simulink model "sampleModel7293"  (R2018a)
settings: Solver=VariableStepAuto  StartTime=0.0  StopTime=10.0  RelTol=1e-3
undefined symbols (not defined in the file): DiscIntNeverNeededParam
libraries: simulink x367
(part 3 of 7)

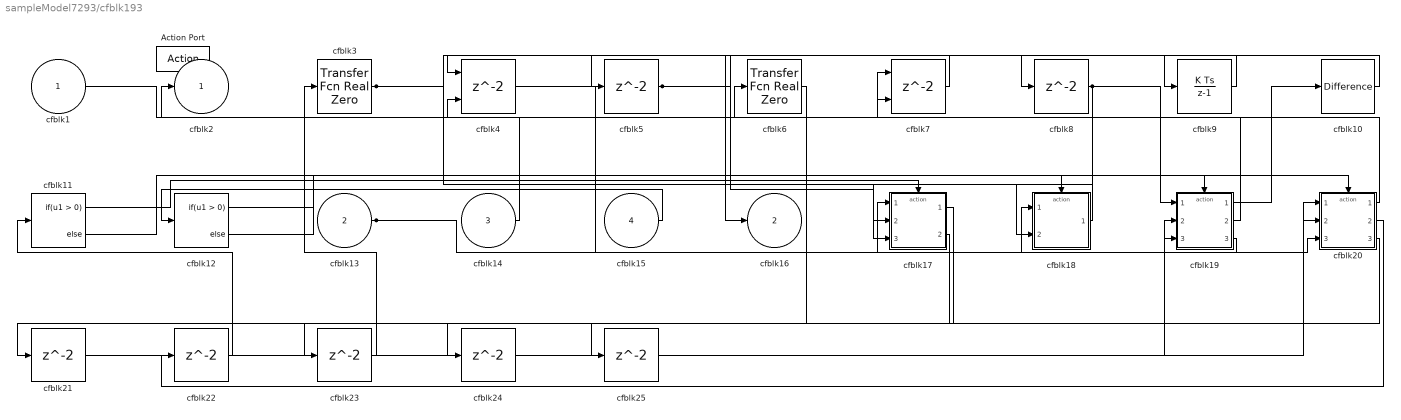
== system sampleModel7293/cfblk193 ==
  cfblk1 : Inport
  cfblk13 : Inport  Port=2
  cfblk14 : Inport  Port=3
  cfblk15 : Inport  Port=4
  Action Port : ActionPort  ActionType=else
  cfblk10 : simulink/Discrete/Difference  ICPrevInput=0.0  OutMin=[]  OutMax=[]  OutDataTypeStr=Inherit: Inherit via back propagation  OutDataType=fixdt(1, 16)  OutScaling=2^-10  DoSatur=off
  cfblk11 : If  SampleTime=1
  cfblk12 : If  SampleTime=1
  cfblk17 : Subsystem  TreatAsAtomicUnit=on
  cfblk18 : Subsystem  TreatAsAtomicUnit=on
  cfblk19 : Subsystem  TreatAsAtomicUnit=on
  cfblk20 : Subsystem  TreatAsAtomicUnit=on
  cfblk{5,8,21..25} (7 alike) : Delay
  cfblk3 : simulink/Discrete/Transfer Fcn Real Zero  ZeroZ=0.75  ICPrevInput=0.0  DoSatur=off
      settings: SourceProductName=Simulink  SourceProductBaseCode=SL
  cfblk4 : Delay  ShowEnablePort=on
      settings: InputPortMap=u0,e6
  cfblk6 : simulink/Discrete/Transfer Fcn Real Zero  ZeroZ=0.75  ICPrevInput=0.0  DoSatur=off
      settings: SourceProductName=Simulink  SourceProductBaseCode=SL
  cfblk7 : Delay  ShowEnablePort=on
      settings: InputPortMap=u0,e6
  cfblk9 : DiscreteIntegrator  SampleTime=-1  ICPrevOutput=DiscIntNeverNeededParam  ICPrevScaledInput=DiscIntNeverNeededParam
  cfblk2 : Outport
  cfblk16 : Outport  Port=2
  wires:
  cfblk18/1(cfblk2) -> cfblk6/1
  cfblk7/1 -> cfblk16/1
  cfblk9/1 -> cfblk4/1
  cfblk19/1(cfblk2) -> cfblk10/1
  cfblk20/1(cfblk2) -> cfblk7/1
  cfblk14/1 -> cfblk4/2
  cfblk4/1 -> cfblk17/1(cfblk1)
  cfblk10/1 -> cfblk9/1
  cfblk5/1 -> cfblk8/1, cfblk17/2(cfblk12)
  cfblk15/1 -> cfblk12/1
  cfblk19/2(cfblk15) -> cfblk2/1
  cfblk1/1 -> cfblk7/2
  cfblk8/1 -> cfblk19/1(cfblk1), cfblk17/3(cfblk13)
  cfblk3/1 -> cfblk5/1, cfblk18/2(cfblk11)
  cfblk13/1 -> cfblk19/2(cfblk13), cfblk20/3(cfblk14)
  cfblk19/3(cfblk16) -> cfblk18/1(cfblk1)
  cfblk11/1 -> cfblk17/Action
  cfblk11/2 -> cfblk18/Action
  cfblk12/1 -> cfblk19/Action
  cfblk12/2 -> cfblk20/Action
  cfblk17/1(cfblk2) -> cfblk21/1
  cfblk21/1 -> cfblk20/1(cfblk1)
  cfblk20/2(cfblk15) -> cfblk22/1
  cfblk22/1 -> cfblk11/1
  cfblk6/1 -> cfblk23/1
  cfblk23/1 -> cfblk3/1
  cfblk20/3(cfblk16) -> cfblk24/1
  cfblk24/1 -> cfblk19/3(cfblk14)
  cfblk17/2(cfblk14) -> cfblk25/1
  cfblk25/1 -> cfblk20/2(cfblk13)

== system sampleModel7293/cfblk194 ==
  cfblk1 : Inport
  Action Port : ActionPort  ActionType=then
  cfblk3 : Delay
  cfblk4 : simulink/Continuous/PID Controller  Controller=PID  TimeDomain=Discrete-time  SampleTime=-1  IntegratorMethod=Forward Euler  FilterMethod=Forward Euler  Form=Parallel  UseFilter=on  ControllerParametersSource=internal  P=1  I=1  D=0  N=100  InitialConditionSource=internal  InitialConditionForIntegrator=0  InitialConditionForFilter=0  ExternalReset=none  LimitOutput=off  UpperSaturationLimit=inf  LowerSaturationLimit=-inf  LinearizeAsGain=off  AntiWindupMode=none  Kb=1  TrackingMode=off  Kt=1  PParamMin=[]  PParamMax=[]  IParamMin=[]  IParamMax=[]  DParamMin=[]  DParamMax=[]  NParamMin=[]  NParamMax=[]  KbParamMin=[]  KbParamMax=[]  KtParamMin=[]  KtParamMax=[]  POutMin=[]  POutMax=[]  IOutMin=[]  IOutMax=[]  DOutMin=[]  DOutMax=[]  NOutMin=[]  NOutMax=[]  KbOutMin=[]  KbOutMax=[]  KtOutMin=[]  KtOutMax=[]  IntegratorOutMin=[]  IntegratorOutMax=[]  FilterOutMin=[]  FilterOutMax=[]  SumOutMin=[]  SumOutMax=[]  SumI1OutMin=[]  SumI1OutMax=[]  SumI2OutMin=[]  SumI2OutMax=[]  SumI3OutMin=[]  SumI3OutMax=[]  SumDOutMin=[]  SumDOutMax=[]  SaturationOutMin=[]  SaturationOutMax=[]  IntegratorContinuousStateAttributes=''  IntegratorStateMustResolveToSignalObject=off  IntegratorRTWStateStorageClass=Auto  FilterContinuousStateAttributes=''  FilterStateMustResolveToSignalObject=off  FilterRTWStateStorageClass=Auto  DifferentiatorICPrevScaledInput=0  DifferentiatorOutMin=[]  DifferentiatorOutMax=[]  InitialConditionSetting=State (most efficient)
  cfblk5 : UnitDelay  SampleTime=-1
  cfblk6 : DiscreteTransferFcn
  cfblk7 : Delay  ShowEnablePort=on
      settings: InputPortMap=u0,e6
  cfblk8 : Delay
  cfblk2 : Outport
  wires:
  cfblk4/1 -> cfblk2/1
  cfblk3/1 -> cfblk6/1
  cfblk1/1 -> cfblk5/1
  cfblk6/1 -> cfblk7/2, cfblk8/1
  cfblk5/1 -> cfblk7/1
  cfblk7/1 -> cfblk4/1
  cfblk8/1 -> cfblk3/1

== system sampleModel7293/cfblk195 ==
  cfblk1 : Inport
  cfblk7 : Inport  Port=2
  Action Port : ActionPort  ActionType=else
  cfblk{10..13} (4 alike) : Delay
  cfblk3 : Delay  ShowEnablePort=on
      settings: InputPortMap=u0,e6
  cfblk4 : simulink/Discrete/Difference  ICPrevInput=0.0  OutMin=[]  OutMax=[]  OutDataTypeStr=Inherit: Inherit via back propagation  OutDataType=fixdt(1, 16)  OutScaling=2^-10  DoSatur=off
  cfblk5 : simulink/Discrete/Transfer Fcn Lead or Lag  PoleZ=0.95  ZeroZ=0.75  ICPrevOutput=0.0  ICPrevInput=0.0  DoSatur=off
      settings: SourceProductName=Simulink  SourceProductBaseCode=SL
  cfblk6 : If  SampleTime=1
  cfblk8 : Subsystem  TreatAsAtomicUnit=on
  cfblk9 : Subsystem  TreatAsAtomicUnit=on
  cfblk2 : Outport
  wires:
  cfblk3/1 -> cfblk5/1, cfblk13/1
  cfblk9/1(cfblk2) -> cfblk8/1(cfblk1)
  cfblk5/1 -> cfblk2/1
  cfblk8/1(cfblk2) -> cfblk4/1, cfblk10/1, cfblk12/1
  cfblk9/2(cfblk14) -> cfblk8/2(cfblk11)
  cfblk7/1 -> cfblk3/1
  cfblk1/1 -> cfblk9/2(cfblk11)
  cfblk9/3(cfblk15) -> cfblk8/3(cfblk12), cfblk3/2
  cfblk6/1 -> cfblk8/Action
  cfblk6/2 -> cfblk9/Action
  cfblk10/1 -> cfblk9/1(cfblk1)
  cfblk4/1 -> cfblk11/1
  cfblk11/1 -> cfblk6/1
  cfblk12/1 -> cfblk9/4(cfblk13)
  cfblk13/1 -> cfblk9/3(cfblk12)

== system sampleModel7293/cfblk196 ==
  cfblk1 : Inport
  cfblk9 : Inport  Port=2
  cfblk10 : Inport  Port=3
  Action Port : ActionPort  ActionType=then
  cfblk11 : Subsystem  TreatAsAtomicUnit=on
  cfblk12 : Subsystem  TreatAsAtomicUnit=on
  cfblk13 : Delay
  cfblk14 : Delay
  cfblk3 : simulink/Continuous/PID Controller  Controller=PID  TimeDomain=Discrete-time  SampleTime=-1  IntegratorMethod=Forward Euler  FilterMethod=Forward Euler  Form=Parallel  UseFilter=on  ControllerParametersSource=internal  P=1  I=1  D=0  N=100  InitialConditionSource=internal  InitialConditionForIntegrator=0  InitialConditionForFilter=0  ExternalReset=none  LimitOutput=off  UpperSaturationLimit=inf  LowerSaturationLimit=-inf  LinearizeAsGain=off  AntiWindupMode=none  Kb=1  TrackingMode=off  Kt=1  PParamMin=[]  PParamMax=[]  IParamMin=[]  IParamMax=[]  DParamMin=[]  DParamMax=[]  NParamMin=[]  NParamMax=[]  KbParamMin=[]  KbParamMax=[]  KtParamMin=[]  KtParamMax=[]  POutMin=[]  POutMax=[]  IOutMin=[]  IOutMax=[]  DOutMin=[]  DOutMax=[]  NOutMin=[]  NOutMax=[]  KbOutMin=[]  KbOutMax=[]  KtOutMin=[]  KtOutMax=[]  IntegratorOutMin=[]  IntegratorOutMax=[]  FilterOutMin=[]  FilterOutMax=[]  SumOutMin=[]  SumOutMax=[]  SumI1OutMin=[]  SumI1OutMax=[]  SumI2OutMin=[]  SumI2OutMax=[]  SumI3OutMin=[]  SumI3OutMax=[]  SumDOutMin=[]  SumDOutMax=[]  SaturationOutMin=[]  SaturationOutMax=[]  IntegratorContinuousStateAttributes=''  IntegratorStateMustResolveToSignalObject=off  IntegratorRTWStateStorageClass=Auto  FilterContinuousStateAttributes=''  FilterStateMustResolveToSignalObject=off  FilterRTWStateStorageClass=Auto  DifferentiatorICPrevScaledInput=0  DifferentiatorOutMin=[]  DifferentiatorOutMax=[]  InitialConditionSetting=State (most efficient)
  cfblk4 : simulink/Discrete/Transfer Fcn Lead or Lag  PoleZ=0.95  ZeroZ=0.75  ICPrevOutput=0.0  ICPrevInput=0.0  DoSatur=off
      settings: SourceProductName=Simulink  SourceProductBaseCode=SL
  cfblk5 : Delay  ShowEnablePort=on
      settings: InputPortMap=u0,e6
  cfblk6 : DiscreteStateSpace  SampleTime=-1
  cfblk7 : DiscreteIntegrator  SampleTime=-1  ICPrevOutput=DiscIntNeverNeededParam  ICPrevScaledInput=DiscIntNeverNeededParam
  cfblk8 : If  SampleTime=1
  cfblk2 : Outport
  wires:
  cfblk12/1(cfblk2) -> cfblk2/1
  cfblk3/1 -> cfblk4/1
  cfblk6/1 -> cfblk7/1
  cfblk10/1 -> cfblk3/1
  cfblk12/2(cfblk12) -> cfblk6/1
  cfblk4/1 -> cfblk12/1(cfblk1)
  cfblk9/1 -> cfblk5/1
  cfblk1/1 -> cfblk11/2(cfblk10), cfblk11/3(cfblk11)
  cfblk11/1(cfblk2) -> cfblk5/2
  cfblk8/1 -> cfblk11/Action
  cfblk8/2 -> cfblk12/Action
  cfblk5/1 -> cfblk13/1
  cfblk13/1 -> cfblk8/1
  cfblk7/1 -> cfblk14/1
  cfblk14/1 -> cfblk11/1(cfblk1)

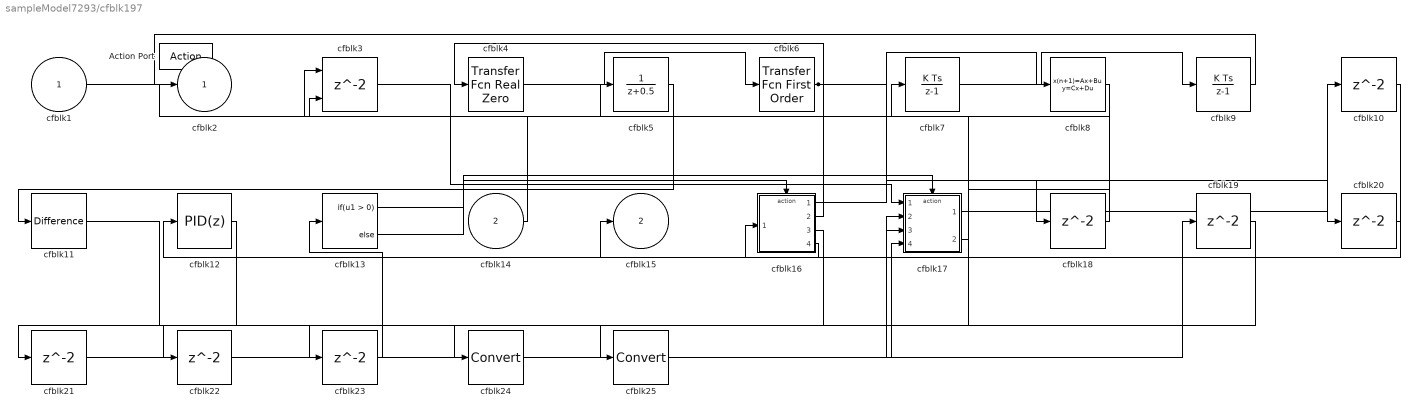
== system sampleModel7293/cfblk197 ==
  cfblk1 : Inport
  cfblk14 : Inport  Port=2
  Action Port : ActionPort  ActionType=else
  cfblk{10,18..23} (7 alike) : Delay
  cfblk11 : simulink/Discrete/Difference  ICPrevInput=0.0  OutMin=[]  OutMax=[]  OutDataTypeStr=Inherit: Inherit via back propagation  OutDataType=fixdt(1, 16)  OutScaling=2^-10  DoSatur=off
  cfblk12 : simulink/Continuous/PID Controller  Controller=PID  TimeDomain=Discrete-time  SampleTime=-1  IntegratorMethod=Forward Euler  FilterMethod=Forward Euler  Form=Parallel  UseFilter=on  ControllerParametersSource=internal  P=1  I=1  D=0  N=100  InitialConditionSource=internal  InitialConditionForIntegrator=0  InitialConditionForFilter=0  ExternalReset=none  LimitOutput=off  UpperSaturationLimit=inf  LowerSaturationLimit=-inf  LinearizeAsGain=off  AntiWindupMode=none  Kb=1  TrackingMode=off  Kt=1  PParamMin=[]  PParamMax=[]  IParamMin=[]  IParamMax=[]  DParamMin=[]  DParamMax=[]  NParamMin=[]  NParamMax=[]  KbParamMin=[]  KbParamMax=[]  KtParamMin=[]  KtParamMax=[]  POutMin=[]  POutMax=[]  IOutMin=[]  IOutMax=[]  DOutMin=[]  DOutMax=[]  NOutMin=[]  NOutMax=[]  KbOutMin=[]  KbOutMax=[]  KtOutMin=[]  KtOutMax=[]  IntegratorOutMin=[]  IntegratorOutMax=[]  FilterOutMin=[]  FilterOutMax=[]  SumOutMin=[]  SumOutMax=[]  SumI1OutMin=[]  SumI1OutMax=[]  SumI2OutMin=[]  SumI2OutMax=[]  SumI3OutMin=[]  SumI3OutMax=[]  SumDOutMin=[]  SumDOutMax=[]  SaturationOutMin=[]  SaturationOutMax=[]  IntegratorContinuousStateAttributes=''  IntegratorStateMustResolveToSignalObject=off  IntegratorRTWStateStorageClass=Auto  FilterContinuousStateAttributes=''  FilterStateMustResolveToSignalObject=off  FilterRTWStateStorageClass=Auto  DifferentiatorICPrevScaledInput=0  DifferentiatorOutMin=[]  DifferentiatorOutMax=[]  InitialConditionSetting=State (most efficient)
  cfblk13 : If  SampleTime=1
  cfblk16 : Subsystem  TreatAsAtomicUnit=on
  cfblk17 : Subsystem  TreatAsAtomicUnit=on
  cfblk24 : DataTypeConversion
  cfblk25 : DataTypeConversion
  cfblk3 : Delay  ShowEnablePort=on
      settings: InputPortMap=u0,e6
  cfblk4 : simulink/Discrete/Transfer Fcn Real Zero  ZeroZ=0.75  ICPrevInput=0.0  DoSatur=off
      settings: SourceProductName=Simulink  SourceProductBaseCode=SL
  cfblk5 : DiscreteTransferFcn
  cfblk6 : simulink/Discrete/Transfer Fcn First Order  PoleZ=0.95  ICPrevOutput=0.0  DoSatur=off
      settings: SourceProductName=Simulink
  cfblk7 : DiscreteIntegrator  SampleTime=-1  ICPrevOutput=DiscIntNeverNeededParam  ICPrevScaledInput=DiscIntNeverNeededParam
  cfblk8 : DiscreteStateSpace  SampleTime=-1
  cfblk9 : DiscreteIntegrator  SampleTime=-1  ICPrevOutput=DiscIntNeverNeededParam  ICPrevScaledInput=DiscIntNeverNeededParam
  cfblk2 : Outport
  cfblk15 : Outport  Port=2
  wires:
  cfblk4/1 -> cfblk6/1
  cfblk7/1 -> cfblk9/1
  cfblk16/2(cfblk11) -> cfblk4/1
  cfblk14/1 -> cfblk3/2
  cfblk10/1 -> cfblk15/1
  cfblk9/1 -> cfblk2/1
  cfblk3/1 -> cfblk17/1(cfblk1)
  cfblk17/1(cfblk2) -> cfblk10/1
  cfblk17/2(cfblk15) -> cfblk5/1
  cfblk1/1 -> cfblk7/1
  cfblk6/1 -> cfblk8/1, cfblk20/1
  cfblk5/1 -> cfblk11/1
  cfblk16/4(cfblk13) -> cfblk12/1
  cfblk13/1 -> cfblk16/Action
  cfblk13/2 -> cfblk17/Action
  cfblk16/1(cfblk2) -> cfblk18/1
  cfblk18/1 -> cfblk3/1
  cfblk20/1 -> cfblk16/1(cfblk1)
  cfblk16/3(cfblk12) -> cfblk21/1
  cfblk21/1 -> cfblk17/4(cfblk14)
  cfblk12/1 -> cfblk22/1
  cfblk22/1 -> cfblk17/3(cfblk13)
  cfblk11/1 -> cfblk23/1
  cfblk23/1 -> cfblk13/1
  cfblk19/1 -> cfblk24/1
  cfblk24/1 -> cfblk17/2(cfblk12)
  cfblk8/1 -> cfblk25/1
  cfblk25/1 -> cfblk19/1

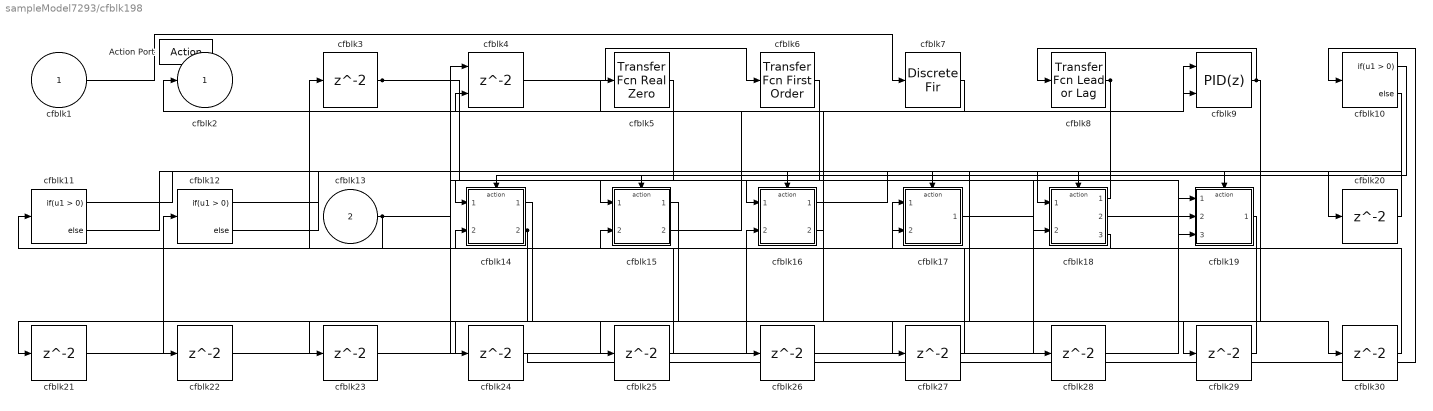
== system sampleModel7293/cfblk198 ==
  cfblk1 : Inport
  cfblk13 : Inport  Port=2
  Action Port : ActionPort  ActionType=then
  cfblk10 : If  SampleTime=1
  cfblk11 : If  SampleTime=1
  cfblk12 : If  SampleTime=1
  cfblk14 : Subsystem  TreatAsAtomicUnit=on
  cfblk15 : Subsystem  TreatAsAtomicUnit=on
  cfblk16 : Subsystem  TreatAsAtomicUnit=on
  cfblk17 : Subsystem  TreatAsAtomicUnit=on
  cfblk18 : Subsystem  TreatAsAtomicUnit=on
  cfblk19 : Subsystem  TreatAsAtomicUnit=on
  cfblk{3,20..30} (12 alike) : Delay
  cfblk4 : Delay  ShowEnablePort=on
      settings: InputPortMap=u0,e6
  cfblk5 : simulink/Discrete/Transfer Fcn Real Zero  ZeroZ=0.75  ICPrevInput=0.0  DoSatur=off
      settings: SourceProductName=Simulink  SourceProductBaseCode=SL
  cfblk6 : simulink/Discrete/Transfer Fcn First Order  PoleZ=0.95  ICPrevOutput=0.0  DoSatur=off
      settings: SourceProductName=Simulink
  cfblk7 : DiscreteFir
  cfblk8 : simulink/Discrete/Transfer Fcn Lead or Lag  PoleZ=0.95  ZeroZ=0.75  ICPrevOutput=0.0  ICPrevInput=0.0  DoSatur=off
      settings: SourceProductName=Simulink  SourceProductBaseCode=SL
  cfblk9 : simulink/Continuous/PID Controller (2DOF)  Controller=PID  TimeDomain=Discrete-time  SampleTime=-1  IntegratorMethod=Forward Euler  FilterMethod=Forward Euler  Form=Parallel  UseFilter=on  ControllerParametersSource=internal  P=1  I=1  D=0  N=100  b=1  c=1  InitialConditionSource=internal  InitialConditionForIntegrator=0  InitialConditionForFilter=0  ExternalReset=none  LimitOutput=off  UpperSaturationLimit=inf  LowerSaturationLimit=-inf  LinearizeAsGain=off  AntiWindupMode=none  Kb=1  TrackingMode=off  Kt=1  PParamMin=[]  PParamMax=[]  IParamMin=[]  IParamMax=[]  DParamMin=[]  DParamMax=[]  NParamMin=[]  NParamMax=[]  bParamMin=[]  bParamMax=[]  cParamMin=[]  cParamMax=[]  KbParamMin=[]  KbParamMax=[]  KtParamMin=[]  KtParamMax=[]  POutMin=[]  POutMax=[]  IOutMin=[]  IOutMax=[]  DOutMin=[]  DOutMax=[]  NOutMin=[]  NOutMax=[]  bOutMin=[]  bOutMax=[]  cOutMin=[]  cOutMax=[]  KbOutMin=[]  KbOutMax=[]  KtOutMin=[]  KtOutMax=[]  IntegratorOutMin=[]  IntegratorOutMax=[]  FilterOutMin=[]  FilterOutMax=[]  SumOutMin=[]  SumOutMax=[]  Sum1OutMin=[]  Sum1OutMax=[]  Sum2OutMin=[]  Sum2OutMax=[]  Sum3OutMin=[]  Sum3OutMax=[]  SumI1OutMin=[]  SumI1OutMax=[]  SumI2OutMin=[]  SumI2OutMax=[]  SumI3OutMin=[]  SumI3OutMax=[]  SumDOutMin=[]  SumDOutMax=[]  SaturationOutMin=[]  SaturationOutMax=[]  IntegratorContinuousStateAttributes=''  IntegratorStateMustResolveToSignalObject=off  IntegratorRTWStateStorageClass=Auto  FilterContinuousStateAttributes=''  FilterStateMustResolveToSignalObject=off  FilterRTWStateStorageClass=Auto  DifferentiatorICPrevScaledInput=0  DifferentiatorOutMin=[]  DifferentiatorOutMax=[]  InitialConditionSetting=State (most efficient)
  cfblk2 : Outport
  wires:
  cfblk7/1 -> cfblk2/1
  cfblk6/1 -> cfblk16/1(cfblk1)
  cfblk4/1 -> cfblk6/1
  cfblk3/1 -> cfblk18/2(cfblk14), cfblk19/3(cfblk10)
  cfblk5/1 -> cfblk14/1(cfblk1)
  cfblk9/1 -> cfblk8/1, cfblk29/1
  cfblk13/1 -> cfblk11/1, cfblk9/2, cfblk15/1(cfblk1)
  cfblk16/2(cfblk15) -> cfblk5/1
  cfblk1/1 -> cfblk7/1
  cfblk15/2(cfblk7) -> cfblk9/1
  cfblk18/1(cfblk2) -> cfblk4/2
  cfblk8/1 -> cfblk26/1, cfblk27/1
  cfblk14/2(cfblk11) -> cfblk23/1, cfblk24/1
  cfblk18/3(cfblk16) -> cfblk17/1(cfblk1)
  cfblk10/1 -> cfblk14/Action
  cfblk10/2 -> cfblk15/Action
  cfblk11/1 -> cfblk16/Action
  cfblk11/2 -> cfblk17/Action
  cfblk12/1 -> cfblk18/Action
  cfblk12/2 -> cfblk19/Action
  cfblk16/1(cfblk2) -> cfblk20/1
  cfblk20/1 -> cfblk18/1(cfblk1)
  cfblk14/1(cfblk2) -> cfblk21/1
  cfblk21/1 -> cfblk12/1
  cfblk19/1(cfblk2) -> cfblk22/1
  cfblk22/1 -> cfblk4/1
  cfblk23/1 -> cfblk16/2(cfblk14)
  cfblk24/1 -> cfblk10/1
  cfblk15/1(cfblk2) -> cfblk25/1
  cfblk25/1 -> cfblk14/2(cfblk10)
  cfblk26/1 -> cfblk19/1(cfblk1)
  cfblk27/1 -> cfblk17/2(cfblk10)
  cfblk17/1(cfblk2) -> cfblk28/1
  cfblk28/1 -> cfblk19/2(cfblk9)
  cfblk29/1 -> cfblk15/2(cfblk6)
  cfblk18/2(cfblk15) -> cfblk30/1
  cfblk30/1 -> cfblk3/1

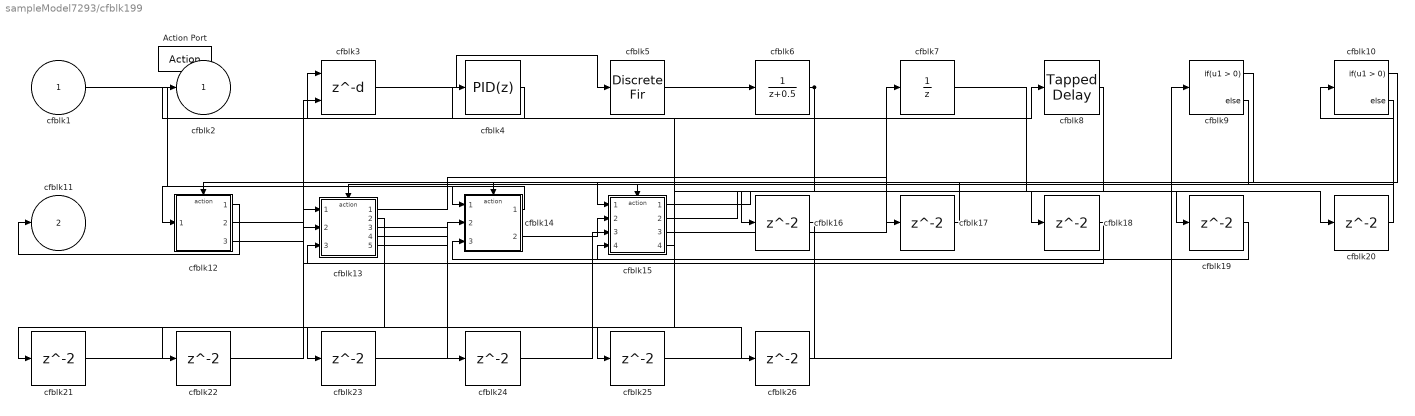
== system sampleModel7293/cfblk199 ==
  cfblk1 : Inport
  Action Port : ActionPort  ActionType=else
  cfblk10 : If  SampleTime=1
  cfblk12 : Subsystem  TreatAsAtomicUnit=on
  cfblk13 : Subsystem  TreatAsAtomicUnit=on
  cfblk14 : Subsystem  TreatAsAtomicUnit=on
  cfblk15 : Subsystem  TreatAsAtomicUnit=on
  cfblk{16..26} (11 alike) : Delay
  cfblk3 : Delay  DelayLengthSource=Input port
      settings: InputPortMap=u0,p1
  cfblk4 : simulink/Continuous/PID Controller  Controller=PID  TimeDomain=Discrete-time  SampleTime=-1  IntegratorMethod=Forward Euler  FilterMethod=Forward Euler  Form=Parallel  UseFilter=on  ControllerParametersSource=internal  P=1  I=1  D=0  N=100  InitialConditionSource=internal  InitialConditionForIntegrator=0  InitialConditionForFilter=0  ExternalReset=none  LimitOutput=off  UpperSaturationLimit=inf  LowerSaturationLimit=-inf  LinearizeAsGain=off  AntiWindupMode=none  Kb=1  TrackingMode=off  Kt=1  PParamMin=[]  PParamMax=[]  IParamMin=[]  IParamMax=[]  DParamMin=[]  DParamMax=[]  NParamMin=[]  NParamMax=[]  KbParamMin=[]  KbParamMax=[]  KtParamMin=[]  KtParamMax=[]  POutMin=[]  POutMax=[]  IOutMin=[]  IOutMax=[]  DOutMin=[]  DOutMax=[]  NOutMin=[]  NOutMax=[]  KbOutMin=[]  KbOutMax=[]  KtOutMin=[]  KtOutMax=[]  IntegratorOutMin=[]  IntegratorOutMax=[]  FilterOutMin=[]  FilterOutMax=[]  SumOutMin=[]  SumOutMax=[]  SumI1OutMin=[]  SumI1OutMax=[]  SumI2OutMin=[]  SumI2OutMax=[]  SumI3OutMin=[]  SumI3OutMax=[]  SumDOutMin=[]  SumDOutMax=[]  SaturationOutMin=[]  SaturationOutMax=[]  IntegratorContinuousStateAttributes=''  IntegratorStateMustResolveToSignalObject=off  IntegratorRTWStateStorageClass=Auto  FilterContinuousStateAttributes=''  FilterStateMustResolveToSignalObject=off  FilterRTWStateStorageClass=Auto  DifferentiatorICPrevScaledInput=0  DifferentiatorOutMin=[]  DifferentiatorOutMax=[]  InitialConditionSetting=State (most efficient)
  cfblk5 : DiscreteFir
  cfblk6 : DiscreteTransferFcn
  cfblk7 : UnitDelay  SampleTime=-1
  cfblk8 : simulink/Discrete/Tapped Delay  vinit=0.0  samptime=-1  NumDelays=1  DelayOrder=Oldest  includeCurrent=off
  cfblk9 : If  SampleTime=1
  cfblk2 : Outport
  cfblk11 : Outport  Port=2
  wires:
  cfblk3/1 -> cfblk5/1
  cfblk1/1 -> cfblk14/1(cfblk1)
  cfblk12/1(cfblk2) -> cfblk11/1
  cfblk5/1 -> cfblk6/1
  cfblk6/1 -> cfblk21/1, cfblk22/1
  cfblk12/2(cfblk9) -> cfblk4/1
  cfblk12/3(cfblk10) -> cfblk8/1
  cfblk4/1 -> cfblk2/1
  cfblk14/1(cfblk2) -> cfblk12/1(cfblk1)
  cfblk15/3(cfblk13) -> cfblk7/1
  cfblk14/2(cfblk7) -> cfblk15/2(cfblk9)
  cfblk15/4(cfblk14) -> cfblk3/1
  cfblk9/1 -> cfblk12/Action
  cfblk9/2 -> cfblk13/Action
  cfblk10/1 -> cfblk14/Action
  cfblk10/2 -> cfblk15/Action
  cfblk8/1 -> cfblk16/1
  cfblk16/1 -> cfblk13/3(cfblk6)
  cfblk13/1(cfblk2) -> cfblk17/1
  cfblk17/1 -> cfblk15/1(cfblk1)
  cfblk15/1(cfblk2) -> cfblk18/1
  cfblk18/1 -> cfblk13/2(cfblk5)
  cfblk15/2(cfblk12) -> cfblk19/1
  cfblk19/1 -> cfblk14/3(cfblk6)
  cfblk7/1 -> cfblk20/1
  cfblk20/1 -> cfblk10/1
  cfblk21/1 -> cfblk13/1(cfblk1)
  cfblk22/1 -> cfblk3/2
  cfblk13/2(cfblk7) -> cfblk23/1
  cfblk23/1 -> cfblk14/2(cfblk5)
  cfblk13/3(cfblk8) -> cfblk24/1
  cfblk24/1 -> cfblk15/3(cfblk10)
  cfblk13/4(cfblk9) -> cfblk25/1
  cfblk25/1 -> cfblk9/1
  cfblk13/5(cfblk10) -> cfblk26/1
  cfblk26/1 -> cfblk15/4(cfblk11)

== system sampleModel7293/cfblk200 ==
  cfblk1 : Inport
  Action Port : ActionPort  ActionType=then
  cfblk10 : If  SampleTime=1
  cfblk11 : Subsystem  TreatAsAtomicUnit=on
  cfblk12 : Subsystem  TreatAsAtomicUnit=on
  cfblk13 : Delay
  cfblk14 : Delay
  cfblk3 : simulink/Discrete/Tapped Delay  vinit=0.0  samptime=-1  NumDelays=1  DelayOrder=Oldest  includeCurrent=off
  cfblk4 : simulink/Discrete/Difference  ICPrevInput=0.0  OutMin=[]  OutMax=[]  OutDataTypeStr=Inherit: Inherit via back propagation  OutDataType=fixdt(1, 16)  OutScaling=2^-10  DoSatur=off
  cfblk5 : Delay  DelayLengthSource=Input port
      settings: InputPortMap=u0,p1
  cfblk6 : Delay
  cfblk7 : UnitDelay  SampleTime=-1
  cfblk8 : simulink/Continuous/PID Controller (2DOF)  Controller=PID  TimeDomain=Discrete-time  SampleTime=-1  IntegratorMethod=Forward Euler  FilterMethod=Forward Euler  Form=Parallel  UseFilter=on  ControllerParametersSource=internal  P=1  I=1  D=0  N=100  b=1  c=1  InitialConditionSource=internal  InitialConditionForIntegrator=0  InitialConditionForFilter=0  ExternalReset=none  LimitOutput=off  UpperSaturationLimit=inf  LowerSaturationLimit=-inf  LinearizeAsGain=off  AntiWindupMode=none  Kb=1  TrackingMode=off  Kt=1  PParamMin=[]  PParamMax=[]  IParamMin=[]  IParamMax=[]  DParamMin=[]  DParamMax=[]  NParamMin=[]  NParamMax=[]  bParamMin=[]  bParamMax=[]  cParamMin=[]  cParamMax=[]  KbParamMin=[]  KbParamMax=[]  KtParamMin=[]  KtParamMax=[]  POutMin=[]  POutMax=[]  IOutMin=[]  IOutMax=[]  DOutMin=[]  DOutMax=[]  NOutMin=[]  NOutMax=[]  bOutMin=[]  bOutMax=[]  cOutMin=[]  cOutMax=[]  KbOutMin=[]  KbOutMax=[]  KtOutMin=[]  KtOutMax=[]  IntegratorOutMin=[]  IntegratorOutMax=[]  FilterOutMin=[]  FilterOutMax=[]  SumOutMin=[]  SumOutMax=[]  Sum1OutMin=[]  Sum1OutMax=[]  Sum2OutMin=[]  Sum2OutMax=[]  Sum3OutMin=[]  Sum3OutMax=[]  SumI1OutMin=[]  SumI1OutMax=[]  SumI2OutMin=[]  SumI2OutMax=[]  SumI3OutMin=[]  SumI3OutMax=[]  SumDOutMin=[]  SumDOutMax=[]  SaturationOutMin=[]  SaturationOutMax=[]  IntegratorContinuousStateAttributes=''  IntegratorStateMustResolveToSignalObject=off  IntegratorRTWStateStorageClass=Auto  FilterContinuousStateAttributes=''  FilterStateMustResolveToSignalObject=off  FilterRTWStateStorageClass=Auto  DifferentiatorICPrevScaledInput=0  DifferentiatorOutMin=[]  DifferentiatorOutMax=[]  InitialConditionSetting=State (most efficient)
  cfblk9 : UnitDelay  SampleTime=-1
  cfblk2 : Outport
  wires:
  cfblk12/1(cfblk2) -> cfblk8/1
  cfblk11/1(cfblk2) -> cfblk4/1
  cfblk1/1 -> cfblk6/1
  cfblk3/1 -> cfblk12/1(cfblk1), cfblk10/1, cfblk8/2
  cfblk7/1 -> cfblk3/1
  cfblk9/1 -> cfblk2/1
  cfblk5/1 -> cfblk7/1, cfblk12/2(cfblk9)
  cfblk6/1 -> cfblk5/2, cfblk9/1
  cfblk10/1 -> cfblk11/Action
  cfblk10/2 -> cfblk12/Action
  cfblk8/1 -> cfblk13/1
  cfblk13/1 -> cfblk5/1
  cfblk4/1 -> cfblk14/1
  cfblk14/1 -> cfblk11/1(cfblk1)

== system sampleModel7293/cfblk201 ==
  cfblk1 : Inport
  Action Port : ActionPort  ActionType=else
  cfblk10 : simulink/Discrete/Transfer Fcn First Order  PoleZ=0.95  ICPrevOutput=0.0  DoSatur=off
      settings: SourceProductName=Simulink
  cfblk11 : DiscreteIntegrator  SampleTime=-1  ICPrevOutput=DiscIntNeverNeededParam  ICPrevScaledInput=DiscIntNeverNeededParam
  cfblk12 : DiscreteTransferFcn
  cfblk13 : simulink/Discrete/Transfer Fcn Real Zero  ZeroZ=0.75  ICPrevInput=0.0  DoSatur=off
      settings: SourceProductName=Simulink  SourceProductBaseCode=SL
  cfblk14 : DiscreteStateSpace  SampleTime=-1
  cfblk15 : Delay
  cfblk3 : UnitDelay  SampleTime=-1
  cfblk4 : Delay  DelayLengthSource=Input port
      settings: InputPortMap=u0,p1
  cfblk5 : DiscreteFir
  cfblk6 : DiscreteTransferFcn
  cfblk7 : DiscreteIntegrator  SampleTime=-1  ICPrevOutput=DiscIntNeverNeededParam  ICPrevScaledInput=DiscIntNeverNeededParam
  cfblk8 : DiscreteStateSpace  SampleTime=-1
  cfblk9 : Delay
  cfblk2 : Outport
  wires:
  cfblk5/1 -> cfblk7/1
  cfblk1/1 -> cfblk5/1, cfblk4/2
  cfblk8/1 -> cfblk14/1
  cfblk11/1 -> cfblk3/1
  cfblk14/1 -> cfblk10/1
  cfblk6/1 -> cfblk12/1
  cfblk13/1 -> cfblk2/1
  cfblk12/1 -> cfblk11/1
  cfblk7/1 -> cfblk6/1
  cfblk3/1 -> cfblk4/1
  cfblk10/1 -> cfblk9/1
  cfblk4/1 -> cfblk13/1
  cfblk9/1 -> cfblk15/1
  cfblk15/1 -> cfblk8/1

== system sampleModel7293/cfblk202 ==
  cfblk1 : Inport
  Action Port : ActionPort  ActionType=then
  cfblk10 : DiscreteStateSpace  SampleTime=-1
  cfblk11 : DiscreteTransferFcn
  cfblk12 : Delay
  cfblk13 : Delay
  cfblk3 : simulink/Discrete/Tapped Delay  vinit=0.0  samptime=-1  NumDelays=1  DelayOrder=Oldest  includeCurrent=off
  cfblk4 : simulink/Discrete/Transfer Fcn Lead or Lag  PoleZ=0.95  ZeroZ=0.75  ICPrevOutput=0.0  ICPrevInput=0.0  DoSatur=off
      settings: SourceProductName=Simulink  SourceProductBaseCode=SL
  cfblk5 : simulink/Continuous/PID Controller (2DOF)  Controller=PID  TimeDomain=Discrete-time  SampleTime=-1  IntegratorMethod=Forward Euler  FilterMethod=Forward Euler  Form=Parallel  UseFilter=on  ControllerParametersSource=internal  P=1  I=1  D=0  N=100  b=1  c=1  InitialConditionSource=internal  InitialConditionForIntegrator=0  InitialConditionForFilter=0  ExternalReset=none  LimitOutput=off  UpperSaturationLimit=inf  LowerSaturationLimit=-inf  LinearizeAsGain=off  AntiWindupMode=none  Kb=1  TrackingMode=off  Kt=1  PParamMin=[]  PParamMax=[]  IParamMin=[]  IParamMax=[]  DParamMin=[]  DParamMax=[]  NParamMin=[]  NParamMax=[]  bParamMin=[]  bParamMax=[]  cParamMin=[]  cParamMax=[]  KbParamMin=[]  KbParamMax=[]  KtParamMin=[]  KtParamMax=[]  POutMin=[]  POutMax=[]  IOutMin=[]  IOutMax=[]  DOutMin=[]  DOutMax=[]  NOutMin=[]  NOutMax=[]  bOutMin=[]  bOutMax=[]  cOutMin=[]  cOutMax=[]  KbOutMin=[]  KbOutMax=[]  KtOutMin=[]  KtOutMax=[]  IntegratorOutMin=[]  IntegratorOutMax=[]  FilterOutMin=[]  FilterOutMax=[]  SumOutMin=[]  SumOutMax=[]  Sum1OutMin=[]  Sum1OutMax=[]  Sum2OutMin=[]  Sum2OutMax=[]  Sum3OutMin=[]  Sum3OutMax=[]  SumI1OutMin=[]  SumI1OutMax=[]  SumI2OutMin=[]  SumI2OutMax=[]  SumI3OutMin=[]  SumI3OutMax=[]  SumDOutMin=[]  SumDOutMax=[]  SaturationOutMin=[]  SaturationOutMax=[]  IntegratorContinuousStateAttributes=''  IntegratorStateMustResolveToSignalObject=off  IntegratorRTWStateStorageClass=Auto  FilterContinuousStateAttributes=''  FilterStateMustResolveToSignalObject=off  FilterRTWStateStorageClass=Auto  DifferentiatorICPrevScaledInput=0  DifferentiatorOutMin=[]  DifferentiatorOutMax=[]  InitialConditionSetting=State (most efficient)
  cfblk6 : UnitDelay  SampleTime=-1
  cfblk7 : DiscreteFir
  cfblk8 : Delay  DelayLengthSource=Input port
      settings: InputPortMap=u0,p1
  cfblk9 : simulink/Continuous/PID Controller (2DOF)  Controller=PID  TimeDomain=Discrete-time  SampleTime=-1  IntegratorMethod=Forward Euler  FilterMethod=Forward Euler  Form=Parallel  UseFilter=on  ControllerParametersSource=internal  P=1  I=1  D=0  N=100  b=1  c=1  InitialConditionSource=internal  InitialConditionForIntegrator=0  InitialConditionForFilter=0  ExternalReset=none  LimitOutput=off  UpperSaturationLimit=inf  LowerSaturationLimit=-inf  LinearizeAsGain=off  AntiWindupMode=none  Kb=1  TrackingMode=off  Kt=1  PParamMin=[]  PParamMax=[]  IParamMin=[]  IParamMax=[]  DParamMin=[]  DParamMax=[]  NParamMin=[]  NParamMax=[]  bParamMin=[]  bParamMax=[]  cParamMin=[]  cParamMax=[]  KbParamMin=[]  KbParamMax=[]  KtParamMin=[]  KtParamMax=[]  POutMin=[]  POutMax=[]  IOutMin=[]  IOutMax=[]  DOutMin=[]  DOutMax=[]  NOutMin=[]  NOutMax=[]  bOutMin=[]  bOutMax=[]  cOutMin=[]  cOutMax=[]  KbOutMin=[]  KbOutMax=[]  KtOutMin=[]  KtOutMax=[]  IntegratorOutMin=[]  IntegratorOutMax=[]  FilterOutMin=[]  FilterOutMax=[]  SumOutMin=[]  SumOutMax=[]  Sum1OutMin=[]  Sum1OutMax=[]  Sum2OutMin=[]  Sum2OutMax=[]  Sum3OutMin=[]  Sum3OutMax=[]  SumI1OutMin=[]  SumI1OutMax=[]  SumI2OutMin=[]  SumI2OutMax=[]  SumI3OutMin=[]  SumI3OutMax=[]  SumDOutMin=[]  SumDOutMax=[]  SaturationOutMin=[]  SaturationOutMax=[]  IntegratorContinuousStateAttributes=''  IntegratorStateMustResolveToSignalObject=off  IntegratorRTWStateStorageClass=Auto  FilterContinuousStateAttributes=''  FilterStateMustResolveToSignalObject=off  FilterRTWStateStorageClass=Auto  DifferentiatorICPrevScaledInput=0  DifferentiatorOutMin=[]  DifferentiatorOutMax=[]  InitialConditionSetting=State (most efficient)
  cfblk2 : Outport
  wires:
  cfblk8/1 -> cfblk9/1
  cfblk3/1 -> cfblk4/1, cfblk9/2, cfblk5/2
  cfblk9/1 -> cfblk2/1
  cfblk6/1 -> cfblk11/1
  cfblk10/1 -> cfblk7/1
  cfblk11/1 -> cfblk5/1, cfblk13/1
  cfblk5/1 -> cfblk8/1
  cfblk1/1 -> cfblk10/1
  cfblk7/1 -> cfblk8/2
  cfblk4/1 -> cfblk12/1
  cfblk12/1 -> cfblk3/1
  cfblk13/1 -> cfblk6/1

== system sampleModel7293/cfblk203 ==
  cfblk1 : Inport
  Action Port : ActionPort  ActionType=else
  cfblk10 : simulink/Discrete/Transfer Fcn Lead or Lag  PoleZ=0.95  ZeroZ=0.75  ICPrevOutput=0.0  ICPrevInput=0.0  DoSatur=off
      settings: SourceProductName=Simulink  SourceProductBaseCode=SL
  cfblk11 : If  SampleTime=1
  cfblk12 : Subsystem  TreatAsAtomicUnit=on
  cfblk13 : Subsystem  TreatAsAtomicUnit=on
  cfblk{6,14..17} (5 alike) : Delay
  cfblk3 : DiscreteIntegrator  SampleTime=-1  ICPrevOutput=DiscIntNeverNeededParam  ICPrevScaledInput=DiscIntNeverNeededParam
  cfblk4 : Delay  ShowEnablePort=on
      settings: InputPortMap=u0,e6
  cfblk5 : simulink/Continuous/PID Controller  Controller=PID  TimeDomain=Discrete-time  SampleTime=-1  IntegratorMethod=Forward Euler  FilterMethod=Forward Euler  Form=Parallel  UseFilter=on  ControllerParametersSource=internal  P=1  I=1  D=0  N=100  InitialConditionSource=internal  InitialConditionForIntegrator=0  InitialConditionForFilter=0  ExternalReset=none  LimitOutput=off  UpperSaturationLimit=inf  LowerSaturationLimit=-inf  LinearizeAsGain=off  AntiWindupMode=none  Kb=1  TrackingMode=off  Kt=1  PParamMin=[]  PParamMax=[]  IParamMin=[]  IParamMax=[]  DParamMin=[]  DParamMax=[]  NParamMin=[]  NParamMax=[]  KbParamMin=[]  KbParamMax=[]  KtParamMin=[]  KtParamMax=[]  POutMin=[]  POutMax=[]  IOutMin=[]  IOutMax=[]  DOutMin=[]  DOutMax=[]  NOutMin=[]  NOutMax=[]  KbOutMin=[]  KbOutMax=[]  KtOutMin=[]  KtOutMax=[]  IntegratorOutMin=[]  IntegratorOutMax=[]  FilterOutMin=[]  FilterOutMax=[]  SumOutMin=[]  SumOutMax=[]  SumI1OutMin=[]  SumI1OutMax=[]  SumI2OutMin=[]  SumI2OutMax=[]  SumI3OutMin=[]  SumI3OutMax=[]  SumDOutMin=[]  SumDOutMax=[]  SaturationOutMin=[]  SaturationOutMax=[]  IntegratorContinuousStateAttributes=''  IntegratorStateMustResolveToSignalObject=off  IntegratorRTWStateStorageClass=Auto  FilterContinuousStateAttributes=''  FilterStateMustResolveToSignalObject=off  FilterRTWStateStorageClass=Auto  DifferentiatorICPrevScaledInput=0  DifferentiatorOutMin=[]  DifferentiatorOutMax=[]  InitialConditionSetting=State (most efficient)
  cfblk7 : Delay  DelayLengthSource=Input port
      settings: InputPortMap=u0,p1
  cfblk8 : simulink/Continuous/PID Controller  Controller=PID  TimeDomain=Discrete-time  SampleTime=-1  IntegratorMethod=Forward Euler  FilterMethod=Forward Euler  Form=Parallel  UseFilter=on  ControllerParametersSource=internal  P=1  I=1  D=0  N=100  InitialConditionSource=internal  InitialConditionForIntegrator=0  InitialConditionForFilter=0  ExternalReset=none  LimitOutput=off  UpperSaturationLimit=inf  LowerSaturationLimit=-inf  LinearizeAsGain=off  AntiWindupMode=none  Kb=1  TrackingMode=off  Kt=1  PParamMin=[]  PParamMax=[]  IParamMin=[]  IParamMax=[]  DParamMin=[]  DParamMax=[]  NParamMin=[]  NParamMax=[]  KbParamMin=[]  KbParamMax=[]  KtParamMin=[]  KtParamMax=[]  POutMin=[]  POutMax=[]  IOutMin=[]  IOutMax=[]  DOutMin=[]  DOutMax=[]  NOutMin=[]  NOutMax=[]  KbOutMin=[]  KbOutMax=[]  KtOutMin=[]  KtOutMax=[]  IntegratorOutMin=[]  IntegratorOutMax=[]  FilterOutMin=[]  FilterOutMax=[]  SumOutMin=[]  SumOutMax=[]  SumI1OutMin=[]  SumI1OutMax=[]  SumI2OutMin=[]  SumI2OutMax=[]  SumI3OutMin=[]  SumI3OutMax=[]  SumDOutMin=[]  SumDOutMax=[]  SaturationOutMin=[]  SaturationOutMax=[]  IntegratorContinuousStateAttributes=''  IntegratorStateMustResolveToSignalObject=off  IntegratorRTWStateStorageClass=Auto  FilterContinuousStateAttributes=''  FilterStateMustResolveToSignalObject=off  FilterRTWStateStorageClass=Auto  DifferentiatorICPrevScaledInput=0  DifferentiatorOutMin=[]  DifferentiatorOutMax=[]  InitialConditionSetting=State (most efficient)
  cfblk9 : Delay  ShowEnablePort=on
      settings: InputPortMap=u0,e6
  cfblk2 : Outport
  wires:
  cfblk5/1 -> cfblk7/1, cfblk11/1
  cfblk9/1 -> cfblk12/1(cfblk1)
  cfblk12/1(cfblk2) -> cfblk10/1, cfblk4/1
  cfblk8/1 -> cfblk13/2(cfblk12)
  cfblk7/1 -> cfblk8/1, cfblk9/2, cfblk4/2
  cfblk1/1 -> cfblk5/1
  cfblk4/1 -> cfblk6/1
  cfblk13/1(cfblk2) -> cfblk3/1
  cfblk13/2(cfblk14) -> cfblk2/1
  cfblk11/1 -> cfblk12/Action
  cfblk11/2 -> cfblk13/Action
  cfblk3/1 -> cfblk14/1
  cfblk14/1 -> cfblk13/3(cfblk13)
  cfblk13/3(cfblk15) -> cfblk15/1
  cfblk15/1 -> cfblk7/2
  cfblk10/1 -> cfblk16/1
  cfblk16/1 -> cfblk13/1(cfblk1)
  cfblk6/1 -> cfblk17/1
  cfblk17/1 -> cfblk9/1

== system sampleModel7293/cfblk204 ==
  cfblk1 : Inport
  cfblk11 : Inport  Port=2
  Action Port : ActionPort  ActionType=then
  cfblk10 : simulink/Discrete/Tapped Delay  vinit=0.0  samptime=-1  NumDelays=1  DelayOrder=Oldest  includeCurrent=off
  cfblk3 : simulink/Discrete/Transfer Fcn Real Zero  ZeroZ=0.75  ICPrevInput=0.0  DoSatur=off
      settings: SourceProductName=Simulink  SourceProductBaseCode=SL
  cfblk4 : simulink/Discrete/Transfer Fcn Lead or Lag  PoleZ=0.95  ZeroZ=0.75  ICPrevOutput=0.0  ICPrevInput=0.0  DoSatur=off
      settings: SourceProductName=Simulink  SourceProductBaseCode=SL
  cfblk5 : DiscreteZeroPole  Poles=[0 0.5]  Gain=1  SampleTime=-1
  cfblk6 : DiscreteZeroPole  Poles=[0 0.5]  Gain=1  SampleTime=-1
  cfblk7 : simulink/Discrete/Difference  ICPrevInput=0.0  OutMin=[]  OutMax=[]  OutDataTypeStr=Inherit: Inherit via back propagation  OutDataType=fixdt(1, 16)  OutScaling=2^-10  DoSatur=off
  cfblk8 : simulink/Discrete/Transfer Fcn Real Zero  ZeroZ=0.75  ICPrevInput=0.0  DoSatur=off
      settings: SourceProductName=Simulink  SourceProductBaseCode=SL
  cfblk9 : DiscreteFilter
  cfblk2 : Outport
  cfblk12 : Outport  Port=2
  cfblk13 : Outport  Port=3
  wires:
  cfblk8/1 -> cfblk2/1
  cfblk11/1 -> cfblk6/1
  cfblk7/1 -> cfblk5/1
  cfblk1/1 -> cfblk12/1
  cfblk6/1 -> cfblk3/1, cfblk7/1
  cfblk10/1 -> cfblk4/1
  cfblk4/1 -> cfblk8/1
  cfblk3/1 -> cfblk10/1
  cfblk5/1 -> cfblk9/1
  cfblk9/1 -> cfblk13/1

== system sampleModel7293/cfblk205 ==
  cfblk1 : Inport
  cfblk9 : Inport  Port=2
  cfblk10 : Inport  Port=3
  Action Port : ActionPort  ActionType=else
  cfblk13 : Delay
  cfblk3 : DiscreteFir
  cfblk4 : simulink/Discrete/Transfer Fcn Lead or Lag  PoleZ=0.95  ZeroZ=0.75  ICPrevOutput=0.0  ICPrevInput=0.0  DoSatur=off
      settings: SourceProductName=Simulink  SourceProductBaseCode=SL
  cfblk5 : DiscreteZeroPole  Poles=[0 0.5]  Gain=1  SampleTime=-1
  cfblk6 : DiscreteFilter
  cfblk7 : simulink/Continuous/PID Controller (2DOF)  Controller=PID  TimeDomain=Discrete-time  SampleTime=-1  IntegratorMethod=Forward Euler  FilterMethod=Forward Euler  Form=Parallel  UseFilter=on  ControllerParametersSource=internal  P=1  I=1  D=0  N=100  b=1  c=1  InitialConditionSource=internal  InitialConditionForIntegrator=0  InitialConditionForFilter=0  ExternalReset=none  LimitOutput=off  UpperSaturationLimit=inf  LowerSaturationLimit=-inf  LinearizeAsGain=off  AntiWindupMode=none  Kb=1  TrackingMode=off  Kt=1  PParamMin=[]  PParamMax=[]  IParamMin=[]  IParamMax=[]  DParamMin=[]  DParamMax=[]  NParamMin=[]  NParamMax=[]  bParamMin=[]  bParamMax=[]  cParamMin=[]  cParamMax=[]  KbParamMin=[]  KbParamMax=[]  KtParamMin=[]  KtParamMax=[]  POutMin=[]  POutMax=[]  IOutMin=[]  IOutMax=[]  DOutMin=[]  DOutMax=[]  NOutMin=[]  NOutMax=[]  bOutMin=[]  bOutMax=[]  cOutMin=[]  cOutMax=[]  KbOutMin=[]  KbOutMax=[]  KtOutMin=[]  KtOutMax=[]  IntegratorOutMin=[]  IntegratorOutMax=[]  FilterOutMin=[]  FilterOutMax=[]  SumOutMin=[]  SumOutMax=[]  Sum1OutMin=[]  Sum1OutMax=[]  Sum2OutMin=[]  Sum2OutMax=[]  Sum3OutMin=[]  Sum3OutMax=[]  SumI1OutMin=[]  SumI1OutMax=[]  SumI2OutMin=[]  SumI2OutMax=[]  SumI3OutMin=[]  SumI3OutMax=[]  SumDOutMin=[]  SumDOutMax=[]  SaturationOutMin=[]  SaturationOutMax=[]  IntegratorContinuousStateAttributes=''  IntegratorStateMustResolveToSignalObject=off  IntegratorRTWStateStorageClass=Auto  FilterContinuousStateAttributes=''  FilterStateMustResolveToSignalObject=off  FilterRTWStateStorageClass=Auto  DifferentiatorICPrevScaledInput=0  DifferentiatorOutMin=[]  DifferentiatorOutMax=[]  InitialConditionSetting=State (most efficient)
  cfblk8 : DiscreteFilter
  cfblk2 : Outport
  cfblk11 : Outport  Port=2
  cfblk12 : Outport  Port=3
  wires:
  cfblk6/1 -> cfblk8/1
  cfblk7/1 -> cfblk5/1, cfblk3/1
  cfblk10/1 -> cfblk6/1
  cfblk9/1 -> cfblk12/1
  cfblk5/1 -> cfblk2/1
  cfblk8/1 -> cfblk11/1
  cfblk1/1 -> cfblk4/1
  cfblk4/1 -> cfblk7/1
  cfblk3/1 -> cfblk13/1
  cfblk13/1 -> cfblk7/2

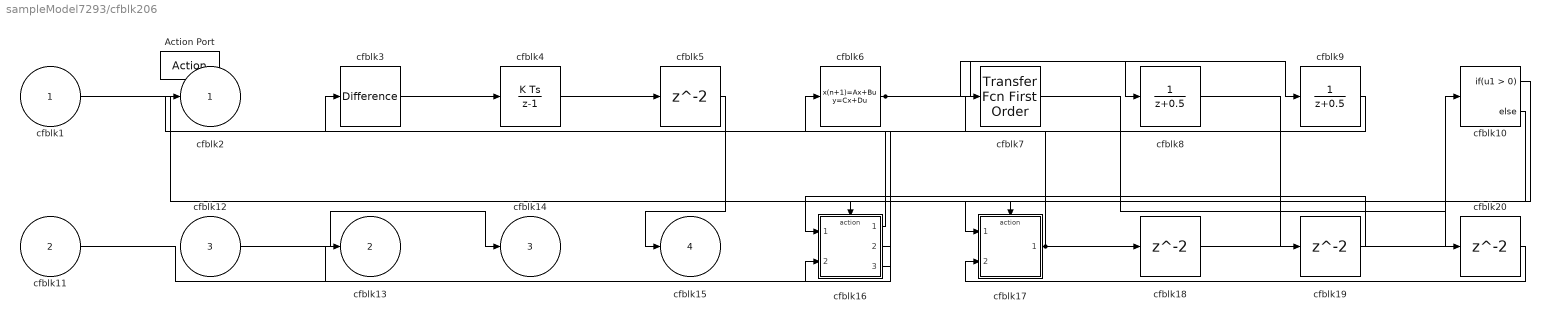
== system sampleModel7293/cfblk206 ==
  cfblk1 : Inport
  cfblk11 : Inport  Port=2
  cfblk12 : Inport  Port=3
  Action Port : ActionPort  ActionType=then
  cfblk10 : If  SampleTime=1
  cfblk16 : Subsystem  TreatAsAtomicUnit=on
  cfblk17 : Subsystem  TreatAsAtomicUnit=on
  cfblk{5,18..20} (4 alike) : Delay
  cfblk3 : simulink/Discrete/Difference  ICPrevInput=0.0  OutMin=[]  OutMax=[]  OutDataTypeStr=Inherit: Inherit via back propagation  OutDataType=fixdt(1, 16)  OutScaling=2^-10  DoSatur=off
  cfblk4 : DiscreteIntegrator  SampleTime=-1  ICPrevOutput=DiscIntNeverNeededParam  ICPrevScaledInput=DiscIntNeverNeededParam
  cfblk6 : DiscreteStateSpace  SampleTime=-1
  cfblk7 : simulink/Discrete/Transfer Fcn First Order  PoleZ=0.95  ICPrevOutput=0.0  DoSatur=off
      settings: SourceProductName=Simulink
  cfblk8 : DiscreteTransferFcn
  cfblk9 : DiscreteTransferFcn
  cfblk2 : Outport
  cfblk13 : Outport  Port=2
  cfblk14 : Outport  Port=3
  cfblk15 : Outport  Port=4
  wires:
  cfblk12/1 -> cfblk14/1
  cfblk6/1 -> cfblk8/1, cfblk9/1
  cfblk1/1 -> cfblk17/1(cfblk1)
  cfblk3/1 -> cfblk4/1
  cfblk9/1 -> cfblk7/1
  cfblk4/1 -> cfblk5/1
  cfblk11/1 -> cfblk16/2(cfblk12)
  cfblk16/1(cfblk2) -> cfblk3/1
  cfblk5/1 -> cfblk15/1
  cfblk16/2(cfblk13) -> cfblk13/1
  cfblk16/3(cfblk14) -> cfblk2/1
  cfblk17/1(cfblk2) -> cfblk6/1, cfblk18/1
  cfblk10/1 -> cfblk16/Action
  cfblk10/2 -> cfblk17/Action
  cfblk18/1 -> cfblk10/1
  cfblk8/1 -> cfblk19/1
  cfblk19/1 -> cfblk16/1(cfblk1)
  cfblk7/1 -> cfblk20/1
  cfblk20/1 -> cfblk17/2(cfblk7)

== system sampleModel7293/cfblk207 ==
  cfblk1 : Inport
  cfblk7 : Inport  Port=2
  Action Port : ActionPort  ActionType=else
  cfblk3 : simulink/Discrete/Transfer Fcn Real Zero  ZeroZ=0.75  ICPrevInput=0.0  DoSatur=off
      settings: SourceProductName=Simulink  SourceProductBaseCode=SL
  cfblk4 : simulink/Discrete/Transfer Fcn Lead or Lag  PoleZ=0.95  ZeroZ=0.75  ICPrevOutput=0.0  ICPrevInput=0.0  DoSatur=off
      settings: SourceProductName=Simulink  SourceProductBaseCode=SL
  cfblk5 : DiscreteFilter
  cfblk6 : UnitDelay  SampleTime=-1
  cfblk2 : Outport
  wires:
  cfblk1/1 -> cfblk3/1
  cfblk4/1 -> cfblk2/1
  cfblk7/1 -> cfblk5/1
  cfblk5/1 -> cfblk4/1
  cfblk3/1 -> cfblk6/1

== system sampleModel7293/cfblk208 ==
  cfblk1 : Inport
  cfblk12 : Inport  Port=2
  Action Port : ActionPort  ActionType=then
  cfblk10 : UnitDelay  SampleTime=-1
  cfblk11 : simulink/Discrete/Transfer Fcn Lead or Lag  PoleZ=0.95  ZeroZ=0.75  ICPrevOutput=0.0  ICPrevInput=0.0  DoSatur=off
      settings: SourceProductName=Simulink  SourceProductBaseCode=SL
  cfblk{8,14..16} (4 alike) : Delay
  cfblk3 : simulink/Continuous/PID Controller (2DOF)  Controller=PID  TimeDomain=Discrete-time  SampleTime=-1  IntegratorMethod=Forward Euler  FilterMethod=Forward Euler  Form=Parallel  UseFilter=on  ControllerParametersSource=internal  P=1  I=1  D=0  N=100  b=1  c=1  InitialConditionSource=internal  InitialConditionForIntegrator=0  InitialConditionForFilter=0  ExternalReset=none  LimitOutput=off  UpperSaturationLimit=inf  LowerSaturationLimit=-inf  LinearizeAsGain=off  AntiWindupMode=none  Kb=1  TrackingMode=off  Kt=1  PParamMin=[]  PParamMax=[]  IParamMin=[]  IParamMax=[]  DParamMin=[]  DParamMax=[]  NParamMin=[]  NParamMax=[]  bParamMin=[]  bParamMax=[]  cParamMin=[]  cParamMax=[]  KbParamMin=[]  KbParamMax=[]  KtParamMin=[]  KtParamMax=[]  POutMin=[]  POutMax=[]  IOutMin=[]  IOutMax=[]  DOutMin=[]  DOutMax=[]  NOutMin=[]  NOutMax=[]  bOutMin=[]  bOutMax=[]  cOutMin=[]  cOutMax=[]  KbOutMin=[]  KbOutMax=[]  KtOutMin=[]  KtOutMax=[]  IntegratorOutMin=[]  IntegratorOutMax=[]  FilterOutMin=[]  FilterOutMax=[]  SumOutMin=[]  SumOutMax=[]  Sum1OutMin=[]  Sum1OutMax=[]  Sum2OutMin=[]  Sum2OutMax=[]  Sum3OutMin=[]  Sum3OutMax=[]  SumI1OutMin=[]  SumI1OutMax=[]  SumI2OutMin=[]  SumI2OutMax=[]  SumI3OutMin=[]  SumI3OutMax=[]  SumDOutMin=[]  SumDOutMax=[]  SaturationOutMin=[]  SaturationOutMax=[]  IntegratorContinuousStateAttributes=''  IntegratorStateMustResolveToSignalObject=off  IntegratorRTWStateStorageClass=Auto  FilterContinuousStateAttributes=''  FilterStateMustResolveToSignalObject=off  FilterRTWStateStorageClass=Auto  DifferentiatorICPrevScaledInput=0  DifferentiatorOutMin=[]  DifferentiatorOutMax=[]  InitialConditionSetting=State (most efficient)
  cfblk4 : UnitDelay  SampleTime=-1
  cfblk5 : DiscreteIntegrator  SampleTime=-1  ICPrevOutput=DiscIntNeverNeededParam  ICPrevScaledInput=DiscIntNeverNeededParam
  cfblk6 : DiscreteStateSpace  SampleTime=-1
  cfblk7 : simulink/Discrete/Transfer Fcn Lead or Lag  PoleZ=0.95  ZeroZ=0.75  ICPrevOutput=0.0  ICPrevInput=0.0  DoSatur=off
      settings: SourceProductName=Simulink  SourceProductBaseCode=SL
  cfblk9 : Delay  DelayLengthSource=Input port
      settings: InputPortMap=u0,p1
  cfblk2 : Outport
  cfblk13 : Outport  Port=2
  wires:
  cfblk6/1 -> cfblk11/1
  cfblk1/1 -> cfblk2/1
  cfblk8/1 -> cfblk9/1
  cfblk12/1 -> cfblk8/1
  cfblk9/1 -> cfblk5/1, cfblk15/1
  cfblk4/1 -> cfblk7/1
  cfblk10/1 -> cfblk9/2
  cfblk3/1 -> cfblk4/1, cfblk13/1
  cfblk7/1 -> cfblk10/1
  cfblk5/1 -> cfblk14/1
  cfblk14/1 -> cfblk3/1
  cfblk15/1 -> cfblk3/2
  cfblk11/1 -> cfblk16/1
  cfblk16/1 -> cfblk6/1

== system sampleModel7293/cfblk209 ==
  cfblk1 : Inport
  Action Port : ActionPort  ActionType=else
  cfblk10 : Subsystem  TreatAsAtomicUnit=on
  cfblk11 : Delay
  cfblk12 : Delay
  cfblk13 : Delay
  cfblk3 : DiscreteTransferFcn
  cfblk4 : DiscreteFir
  cfblk5 : simulink/Continuous/PID Controller (2DOF)  Controller=PID  TimeDomain=Discrete-time  SampleTime=-1  IntegratorMethod=Forward Euler  FilterMethod=Forward Euler  Form=Parallel  UseFilter=on  ControllerParametersSource=internal  P=1  I=1  D=0  N=100  b=1  c=1  InitialConditionSource=internal  InitialConditionForIntegrator=0  InitialConditionForFilter=0  ExternalReset=none  LimitOutput=off  UpperSaturationLimit=inf  LowerSaturationLimit=-inf  LinearizeAsGain=off  AntiWindupMode=none  Kb=1  TrackingMode=off  Kt=1  PParamMin=[]  PParamMax=[]  IParamMin=[]  IParamMax=[]  DParamMin=[]  DParamMax=[]  NParamMin=[]  NParamMax=[]  bParamMin=[]  bParamMax=[]  cParamMin=[]  cParamMax=[]  KbParamMin=[]  KbParamMax=[]  KtParamMin=[]  KtParamMax=[]  POutMin=[]  POutMax=[]  IOutMin=[]  IOutMax=[]  DOutMin=[]  DOutMax=[]  NOutMin=[]  NOutMax=[]  bOutMin=[]  bOutMax=[]  cOutMin=[]  cOutMax=[]  KbOutMin=[]  KbOutMax=[]  KtOutMin=[]  KtOutMax=[]  IntegratorOutMin=[]  IntegratorOutMax=[]  FilterOutMin=[]  FilterOutMax=[]  SumOutMin=[]  SumOutMax=[]  Sum1OutMin=[]  Sum1OutMax=[]  Sum2OutMin=[]  Sum2OutMax=[]  Sum3OutMin=[]  Sum3OutMax=[]  SumI1OutMin=[]  SumI1OutMax=[]  SumI2OutMin=[]  SumI2OutMax=[]  SumI3OutMin=[]  SumI3OutMax=[]  SumDOutMin=[]  SumDOutMax=[]  SaturationOutMin=[]  SaturationOutMax=[]  IntegratorContinuousStateAttributes=''  IntegratorStateMustResolveToSignalObject=off  IntegratorRTWStateStorageClass=Auto  FilterContinuousStateAttributes=''  FilterStateMustResolveToSignalObject=off  FilterRTWStateStorageClass=Auto  DifferentiatorICPrevScaledInput=0  DifferentiatorOutMin=[]  DifferentiatorOutMax=[]  InitialConditionSetting=State (most efficient)
  cfblk6 : simulink/Discrete/Transfer Fcn Lead or Lag  PoleZ=0.95  ZeroZ=0.75  ICPrevOutput=0.0  ICPrevInput=0.0  DoSatur=off
      settings: SourceProductName=Simulink  SourceProductBaseCode=SL
  cfblk7 : simulink/Discrete/Difference  ICPrevInput=0.0  OutMin=[]  OutMax=[]  OutDataTypeStr=Inherit: Inherit via back propagation  OutDataType=fixdt(1, 16)  OutScaling=2^-10  DoSatur=off
  cfblk8 : If  SampleTime=1
  cfblk9 : Subsystem  TreatAsAtomicUnit=on
  cfblk2 : Outport
  wires:
  cfblk9/1(cfblk2) -> cfblk3/1
  cfblk10/1(cfblk2) -> cfblk2/1
  cfblk3/1 -> cfblk5/1
  cfblk6/1 -> cfblk4/1
  cfblk9/2(cfblk16) -> cfblk5/2
  cfblk1/1 -> cfblk6/1
  cfblk4/1 -> cfblk8/1
  cfblk10/2(cfblk13) -> cfblk9/2(cfblk15)
  cfblk10/3(cfblk14) -> cfblk7/1
  cfblk7/1 -> cfblk12/1, cfblk13/1
  cfblk8/1 -> cfblk9/Action
  cfblk8/2 -> cfblk10/Action
  cfblk5/1 -> cfblk11/1
  cfblk11/1 -> cfblk9/1(cfblk1)
  cfblk12/1 -> cfblk10/1(cfblk1)
  cfblk13/1 -> cfblk10/2(cfblk12)

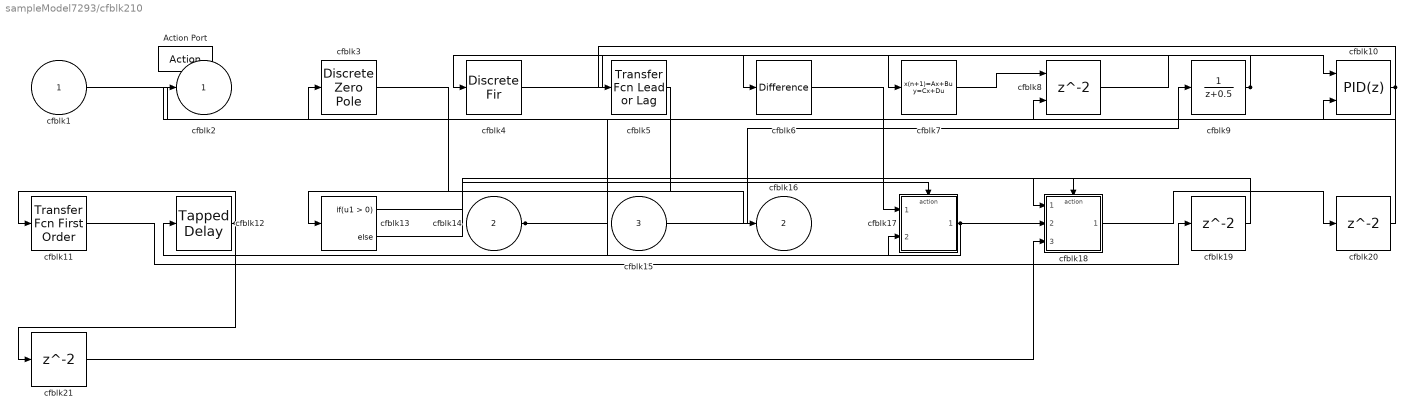
== system sampleModel7293/cfblk210 ==
  cfblk1 : Inport
  cfblk14 : Inport  Port=2
  cfblk15 : Inport  Port=3
  Action Port : ActionPort  ActionType=then
  cfblk10 : simulink/Continuous/PID Controller (2DOF)  Controller=PID  TimeDomain=Discrete-time  SampleTime=-1  IntegratorMethod=Forward Euler  FilterMethod=Forward Euler  Form=Parallel  UseFilter=on  ControllerParametersSource=internal  P=1  I=1  D=0  N=100  b=1  c=1  InitialConditionSource=internal  InitialConditionForIntegrator=0  InitialConditionForFilter=0  ExternalReset=none  LimitOutput=off  UpperSaturationLimit=inf  LowerSaturationLimit=-inf  LinearizeAsGain=off  AntiWindupMode=none  Kb=1  TrackingMode=off  Kt=1  PParamMin=[]  PParamMax=[]  IParamMin=[]  IParamMax=[]  DParamMin=[]  DParamMax=[]  NParamMin=[]  NParamMax=[]  bParamMin=[]  bParamMax=[]  cParamMin=[]  cParamMax=[]  KbParamMin=[]  KbParamMax=[]  KtParamMin=[]  KtParamMax=[]  POutMin=[]  POutMax=[]  IOutMin=[]  IOutMax=[]  DOutMin=[]  DOutMax=[]  NOutMin=[]  NOutMax=[]  bOutMin=[]  bOutMax=[]  cOutMin=[]  cOutMax=[]  KbOutMin=[]  KbOutMax=[]  KtOutMin=[]  KtOutMax=[]  IntegratorOutMin=[]  IntegratorOutMax=[]  FilterOutMin=[]  FilterOutMax=[]  SumOutMin=[]  SumOutMax=[]  Sum1OutMin=[]  Sum1OutMax=[]  Sum2OutMin=[]  Sum2OutMax=[]  Sum3OutMin=[]  Sum3OutMax=[]  SumI1OutMin=[]  SumI1OutMax=[]  SumI2OutMin=[]  SumI2OutMax=[]  SumI3OutMin=[]  SumI3OutMax=[]  SumDOutMin=[]  SumDOutMax=[]  SaturationOutMin=[]  SaturationOutMax=[]  IntegratorContinuousStateAttributes=''  IntegratorStateMustResolveToSignalObject=off  IntegratorRTWStateStorageClass=Auto  FilterContinuousStateAttributes=''  FilterStateMustResolveToSignalObject=off  FilterRTWStateStorageClass=Auto  DifferentiatorICPrevScaledInput=0  DifferentiatorOutMin=[]  DifferentiatorOutMax=[]  InitialConditionSetting=State (most efficient)
  cfblk11 : simulink/Discrete/Transfer Fcn First Order  PoleZ=0.95  ICPrevOutput=0.0  DoSatur=off
      settings: SourceProductName=Simulink
  cfblk12 : simulink/Discrete/Tapped Delay  vinit=0.0  samptime=-1  NumDelays=1  DelayOrder=Oldest  includeCurrent=off
  cfblk13 : If  SampleTime=1
  cfblk17 : Subsystem  TreatAsAtomicUnit=on
  cfblk18 : Subsystem  TreatAsAtomicUnit=on
  cfblk19 : Delay
  cfblk20 : Delay
  cfblk21 : Delay
  cfblk3 : DiscreteZeroPole  Poles=[0 0.5]  Gain=1  SampleTime=-1
  cfblk4 : DiscreteFir
  cfblk5 : simulink/Discrete/Transfer Fcn Lead or Lag  PoleZ=0.95  ZeroZ=0.75  ICPrevOutput=0.0  ICPrevInput=0.0  DoSatur=off
      settings: SourceProductName=Simulink  SourceProductBaseCode=SL
  cfblk6 : simulink/Discrete/Difference  ICPrevInput=0.0  OutMin=[]  OutMax=[]  OutDataTypeStr=Inherit: Inherit via back propagation  OutDataType=fixdt(1, 16)  OutScaling=2^-10  DoSatur=off
  cfblk7 : DiscreteStateSpace  SampleTime=-1
  cfblk8 : Delay  ShowEnablePort=on
      settings: InputPortMap=u0,e6
  cfblk9 : DiscreteTransferFcn
  cfblk2 : Outport
  cfblk16 : Outport  Port=2
  wires:
  cfblk7/1 -> cfblk8/1
  cfblk14/1 -> cfblk8/2, cfblk17/2(cfblk8)
  cfblk4/1 -> cfblk7/1
  cfblk15/1 -> cfblk9/1
  cfblk8/1 -> cfblk10/1
  cfblk17/1(cfblk2) -> cfblk12/1, cfblk18/2(cfblk12)
  cfblk10/1 -> cfblk5/1, cfblk2/1
  cfblk12/1 -> cfblk11/1, cfblk21/1
  cfblk1/1 -> cfblk3/1
  cfblk5/1 -> cfblk13/1
  cfblk9/1 -> cfblk4/1, cfblk6/1
  cfblk3/1 -> cfblk16/1
  cfblk6/1 -> cfblk17/1(cfblk1)
  cfblk13/1 -> cfblk17/Action
  cfblk13/2 -> cfblk18/Action
  cfblk11/1 -> cfblk19/1
  cfblk19/1 -> cfblk18/1(cfblk1)
  cfblk18/1(cfblk2) -> cfblk20/1
  cfblk20/1 -> cfblk10/2
  cfblk21/1 -> cfblk18/3(cfblk13)

== system sampleModel7293/cfblk211 ==
  cfblk1 : Inport
  Action Port : ActionPort  ActionType=else
  cfblk3 : DiscreteTransferFcn
  cfblk4 : Delay
  cfblk5 : simulink/Discrete/Transfer Fcn First Order  PoleZ=0.95  ICPrevOutput=0.0  DoSatur=off
      settings: SourceProductName=Simulink
  cfblk8 : Delay
  cfblk2 : Outport
  cfblk6 : Outport  Port=2
  cfblk7 : Outport  Port=3
  wires:
  cfblk3/1 -> cfblk2/1
  cfblk1/1 -> cfblk6/1
  cfblk5/1 -> cfblk7/1, cfblk8/1
  cfblk4/1 -> cfblk5/1, cfblk3/1
  cfblk8/1 -> cfblk4/1
